simulink model "fixedPoint_model_q3_b"  (R2020b)
settings: Solver=FixedStepDiscrete  StartTime=0.0  StopTime=10  FixedStep=1/44100  RelTol=1e-3  EnableMultiTasking=on
libraries: dspvision x1
settings Model: SILPILModeSetting=veronly  ExtModeTrigDuration=2  Creator=Faridodin  LastModifiedBy=Faridodin
settings RTWCC: BuildConfiguration=Faster Runs

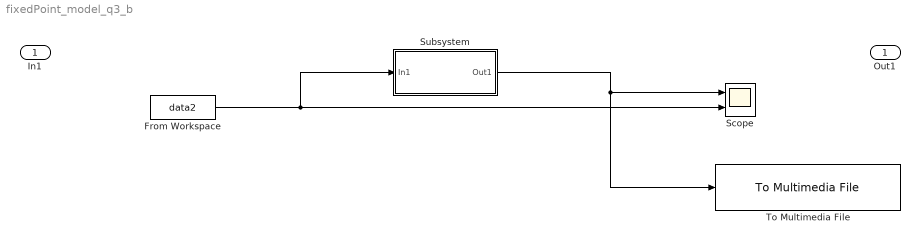
== system fixedPoint_model_q3_b ==
  In1 : Inport
  From Workspace : FromWorkspace  VariableName=data2  SampleTime=-1
  Scope : Scope  NumInputPorts=2
  Subsystem : Subsystem
  To Multimedia File : dspvision/To Multimedia File  outputFilename=outputResult.wav  streamSelection=Audio only  videoCompressor=None (uncompressed)  audioCompressor=None (uncompressed)  imagePorts=Separate color signals  fileType=WAV  audioDatatype=16-bit integer  fourcc=RGB  videoQuality=75  mj2000CompFactor=10
  Out1 : Outport
  wires:
  From Workspace/1 -> Subsystem/1(In1), Scope/2
  Subsystem/1(Out1) -> To Multimedia File/1, Scope/1

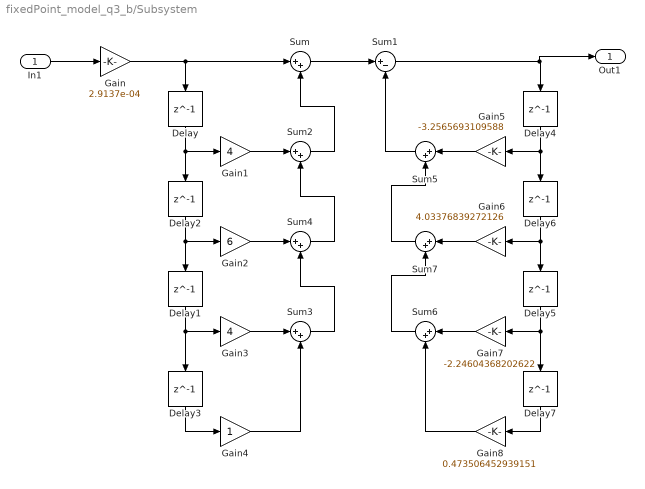
== system fixedPoint_model_q3_b/Subsystem ==
  In1 : Inport
  Delay{,1..7} (8 alike) : Delay  DelayLength=1  InitialCondition=0
  Gain : Gain  Gain=2.9137e-04
  Gain1 : Gain  Gain=4
  Gain2 : Gain  Gain=6
  Gain3 : Gain  Gain=4
  Gain4 : Gain
  Gain5 : Gain  Gain=-3.2565693109588
  Gain6 : Gain  Gain=4.03376839272126
  Gain7 : Gain  Gain=-2.24604368202622
  Gain8 : Gain  Gain=0.473506452939151
  Sum{,2..7} (7 alike) : Sum  Inputs=|++
  Sum1 : Sum  Inputs=|+-
  Out1 : Outport
  wires:
  Delay4/1 -> Delay6/1, Gain5/1
  Gain4/1 -> Sum3/2
  Sum5/1 -> Sum1/2
  Sum3/1 -> Sum4/2
  Delay7/1 -> Gain8/1
  Delay/1 -> Delay2/1, Gain1/1
  Delay3/1 -> Gain4/1
  Delay1/1 -> Delay3/1, Gain3/1
  Gain3/1 -> Sum3/1
  Sum1/1 -> Out1/1, Delay4/1
  Gain8/1 -> Sum6/2
  Gain7/1 -> Sum6/1
  Gain6/1 -> Sum7/1
  Sum6/1 -> Sum7/2
  Delay6/1 -> Delay5/1, Gain6/1
  Sum/1 -> Sum1/1
  Gain5/1 -> Sum5/1
  Delay2/1 -> Delay1/1, Gain2/1
  Sum4/1 -> Sum2/2
  Sum7/1 -> Sum5/2
  Gain2/1 -> Sum4/1
  Gain/1 -> Sum/1, Delay/1
  Sum2/1 -> Sum/2
  Gain1/1 -> Sum2/1
  Delay5/1 -> Delay7/1, Gain7/1
  In1/1 -> Gain/1
